simulink model "PulseGenerator"  (R2024b)
settings: Solver=ode45  StartTime=0.0  StopTime=0.01  MaxStep=1e-7  RelTol=1e-3
undefined symbols (not defined in the file): Tsw
libraries: spsTriangleGeneratorLib x1
settings Model: Creator=ykamatan  LastModifiedBy=ykamatan
settings SolverCC: AlgebraicLoopSolver=TrustRegion
settings DebuggingCC: UnconnectedInputMsg=warning  UnconnectedOutputMsg=warning  UnconnectedLineMsg=warning  ArithmeticOperatorsInVariantConditions=warning
settings ModelReferenceCC: EnableRefExpFcnMdlSchedulingChecks=on
settings SFSimCC: SimUseLocalCustomCode=off  CustomCodeUndefinedFunction=UseInterfaceOnly
settings RTWCC: RTWUseLocalCustomCode=off  GPUComputeCapability=3.5  DLArmComputeVersion=19.05
settings CodeAppCC: StateflowObjectComments=on
settings SimscapeCC: SimscapeNormalizeSystem=off

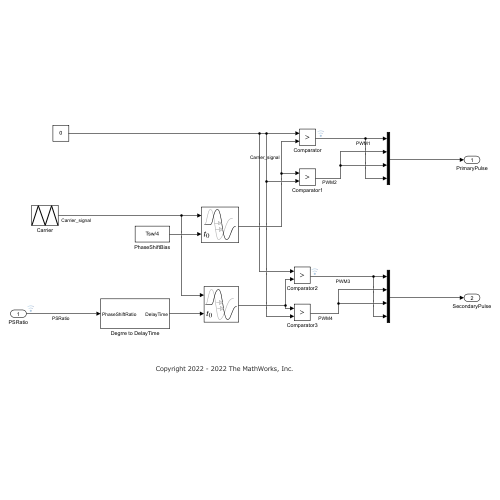
[thumbnail: Simulink's stored preview of the top-level diagram]
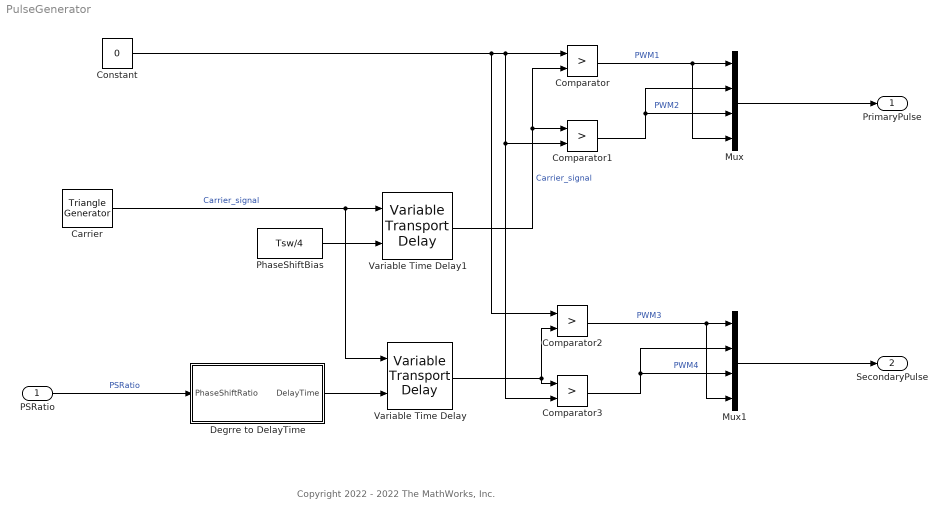
== system PulseGenerator ==
  note: Copyright 2022 - 2022 The MathWorks, Inc.
  PSRatio : Inport
  Carrier : spsTriangleGeneratorLib/Triangle Generator  Freq=Fsw  Phase=0  Ts=0
  Comparator{,1..3} (4 alike) : RelationalOperator  Operator=>  OutDataTypeStr=boolean  RndMeth=Simplest  InputSameDT=off
  Constant : Constant  Value=0
  Degrre to DelayTime : Subsystem
  Mux : Mux
  Mux1 : Mux
  PhaseShiftBias : Constant  Value=Tsw/4
  Variable Time Delay : VariableTransportDelay  MaximumDelay=Tsw  ZeroDelay=on  PadeOrder=3
  Variable Time Delay1 : VariableTransportDelay  MaximumDelay=Tsw  ZeroDelay=on  PadeOrder=3
  PrimaryPulse : Outport
  SecondaryPulse : Outport  Port=2
  wires:
  Variable Time Delay1/1 -> Comparator1/1, Comparator/2  "Carrier_signal"
  Constant/1 -> Comparator1/2, Comparator3/2, Comparator/1, Comparator2/1
  Comparator/1 -> Mux/4, Mux/1  "PWM1"
  Comparator1/1 -> Mux/2, Mux/3  "PWM2"
  Mux/1 -> PrimaryPulse/1
  Comparator2/1 -> Mux1/4, Mux1/1  "PWM3"
  Comparator3/1 -> Mux1/3, Mux1/2  "PWM4"
  Mux1/1 -> SecondaryPulse/1
  Variable Time Delay/1 -> Comparator3/1, Comparator2/2
  Carrier/1 -> Variable Time Delay/1, Variable Time Delay1/1  "Carrier_signal"
  PhaseShiftBias/1 -> Variable Time Delay1/2
  PSRatio/1 -> Degrre to DelayTime/1(PhaseShiftRatio)  "PSRatio"
  Degrre to DelayTime/1(DelayTime) -> Variable Time Delay/2

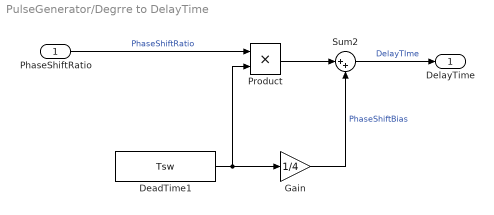
== system PulseGenerator/Degrre to DelayTime ==
  PhaseShiftRatio : Inport
  DeadTime1 : Constant  Value=Tsw
  Gain : Gain  Gain=1/4
  Product : Product
  Sum2 : Sum  Inputs=|++
  DelayTime : Outport
  wires:
  PhaseShiftRatio/1 -> Product/1  "PhaseShiftRatio"
  Sum2/1 -> DelayTime/1  "DelayTIme"
  Gain/1 -> Sum2/2  "PhaseShiftBias"
  DeadTime1/1 -> Product/2, Gain/1
  Product/1 -> Sum2/1
